simulink model "analogtodigital"  (R2022b)
settings: Solver=VariableStepAuto  StartTime=0.0  StopTime=T  MaxStep=MaxStep  RelTol=RelTol
values from neighbouring files (symbols this model uses):
  J = 20    [initialization.m]
  T = 10    [initialization.m]
libraries: HyEQ_Library x1
settings Model: Creator=tom  LastModifiedBy=tom

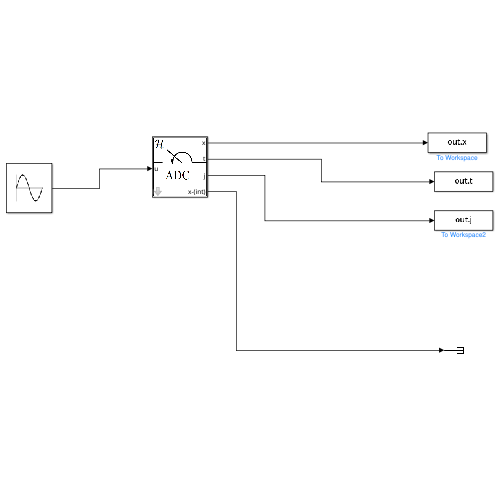
[thumbnail: Simulink's stored preview of the top-level diagram]
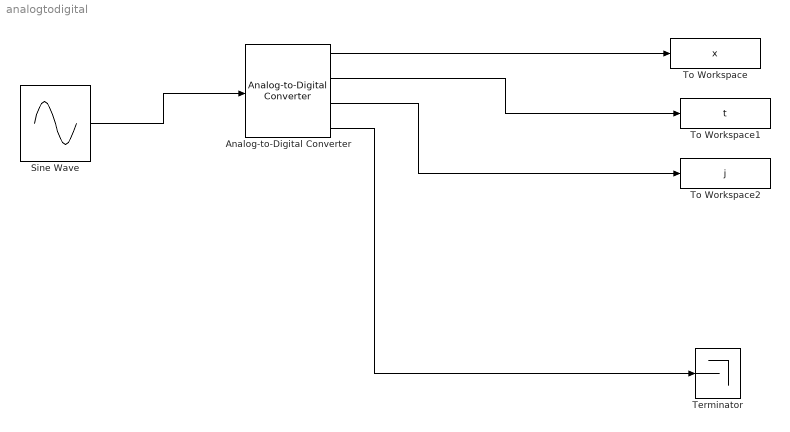
== system analogtodigital ==
  Analog-to-Digital Converter : HyEQ_Library/Cyber Physical Systems/Analog-to-Digital Converter  sample_time=Ts  u0=0  tau0=0  T=T  J=J
      settings: SourceProductName=Hybrid Equations Toolbox
  Sine Wave : Sin  SampleTime=0
  Terminator : Terminator
  To Workspace : ToWorkspace  VariableName=x  SaveFormat=Timeseries  SampleTime=-1
  To Workspace1 : ToWorkspace  VariableName=t  SaveFormat=Timeseries  SampleTime=-1
  To Workspace2 : ToWorkspace  VariableName=j  SaveFormat=Timeseries  SampleTime=-1
  wires:
  Sine Wave/1 -> Analog-to-Digital Converter/1
  Analog-to-Digital Converter/1 -> To Workspace/1
  Analog-to-Digital Converter/2 -> To Workspace1/1
  Analog-to-Digital Converter/3 -> To Workspace2/1
  Analog-to-Digital Converter/4 -> Terminator/1
